simulink model "control1_flatness"  (R2023b)
settings: Solver=VariableStepAuto  StartTime=0.0  StopTime=8  RelTol=1e-3
values from neighbouring files (symbols this model uses):
  d = obs_r+threshold    (= 0.3)    [main.m]
  damping_coeff = 1/sqrt(2)    [main.m]
  initial_position = [0,r]    [main.m]
  natural_frequency = 10    [main.m]
  obs_r = 0.1    [main.m]
  obs_x = [20]    [main.m]
  obs_y = [20]    [main.m]
  parking_position = [0,0]    [main.m]
  r = 1    [main.m]
  T = 2*pi    (= 6.28318530718)    [main.m]
  t_values = 0:dt:T*1.1    [main.m]
  threshold = 0.2    [main.m]
(part 2 of 3)

== system control1_flatness/Trajectory generator/Trajectory generator and obstacle detection2/Subsystem3 ==
  Enable : EnablePort
  Clock1 : Clock
  Constant3 : Constant  Value=t_values
  Data Store Read : DataStoreRead  DataStoreName=iteration  IndexOptions=Index vector (dialog)  Indices=1  OutputSizes=1
  Data Store Read11 : DataStoreRead  DataStoreName=trajectory_x  IndexOptions=Index vector (dialog)  Indices=1  OutputSizes=1
  Data Store Read12 : DataStoreRead  DataStoreName=trajectory_y  IndexOptions=Index vector (dialog)  Indices=1  OutputSizes=1
  Data Store Read13 : DataStoreRead  DataStoreName=v_d_array  IndexOptions=Index vector (dialog)  Indices=1  OutputSizes=1
  Data Store Read14 : DataStoreRead  DataStoreName=omega_d_array  IndexOptions=Index vector (dialog)  Indices=1  OutputSizes=1
  Data Store Read15 : DataStoreRead  DataStoreName=theta_d_array  IndexOptions=Index vector (dialog)  Indices=1  OutputSizes=1
  Data Store Write : DataStoreWrite  DataStoreName=iteration  IndexOptions=Index vector (dialog)  Indices=1  OutputSizes=1
  Triggered Subsystem : Subsystem  TreatAsAtomicUnit=on
  x_d : Outport
  y_d : Outport  Port=2
  v_d : Outport  Port=3
  omega_d : Outport  Port=4
  theta_d : Outport  Port=5
  new_i : Outport  Port=6
  wires:
  Triggered Subsystem/3(v_d) -> v_d/1
  Triggered Subsystem/1(x_d) -> x_d/1
  Triggered Subsystem/2(y_d) -> y_d/1
  Data Store Read12/1 -> Triggered Subsystem/4(trajectory_y)
  Triggered Subsystem/4(omega_d) -> omega_d/1
  Data Store Read15/1 -> Triggered Subsystem/7(theta_d_array)
  Data Store Read14/1 -> Triggered Subsystem/6(omega_d_array)
  Data Store Read11/1 -> Triggered Subsystem/3(trajectory_x)
  Data Store Read13/1 -> Triggered Subsystem/5(v_d_array)
  Triggered Subsystem/5(theta_d) -> theta_d/1
  Clock1/1 -> Triggered Subsystem/1(t)
  Constant3/1 -> Triggered Subsystem/2(t_values)
  Data Store Read/1 -> Triggered Subsystem/8(Input)
  Triggered Subsystem/6(new_i) -> Data Store Write/1, new_i/1

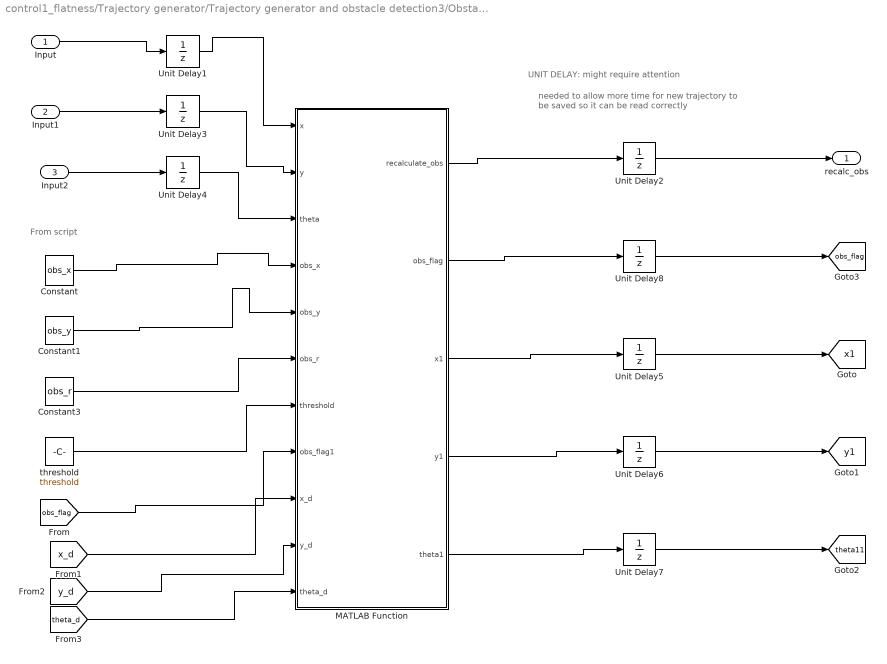
== system control1_flatness/Trajectory generator/Trajectory generator and obstacle detection3/Obstacle Detection ==
  note: UNIT DELAY: might require attention
  note: needed to allow more time for new trajectory to be saved
      | so it can be read correctly
  note: From script
  Input : Inport
  Input1 : Inport  Port=2
  Input2 : Inport  Port=3
  Constant : Constant  Value=obs_x
  Constant1 : Constant  Value=obs_y
  Constant3 : Constant  Value=obs_r
  MATLAB Function : MATLAB Function  TreatAsAtomicUnit=on
  Unit Delay{1..8} (8 alike) : UnitDelay  SampleTime=0.001  HasFrameUpgradeWarning=on
  threshold : Constant  Value=threshold
  recalc_obs : Outport
  tag scope: obs_flag=global, theta11=global, x1=global, y1=global
  wires:
  Constant/1 -> MATLAB Function/4(obs_x)
  Constant1/1 -> MATLAB Function/5(obs_y)
  Constant3/1 -> MATLAB Function/6(obs_r)
  threshold/1 -> MATLAB Function/7(threshold)
  [obs_flag] -> MATLAB Function/8(obs_flag1)
  MATLAB Function/2(obs_flag) -> Unit Delay8/1
  MATLAB Function/1(recalculate_obs) -> Unit Delay2/1
  Input/1 -> Unit Delay1/1
  Input1/1 -> Unit Delay3/1
  Unit Delay2/1 -> recalc_obs/1
  Unit Delay1/1 -> MATLAB Function/1(x)
  Unit Delay3/1 -> MATLAB Function/2(y)
  Input2/1 -> Unit Delay4/1
  Unit Delay4/1 -> MATLAB Function/3(theta)
  MATLAB Function/3(x1) -> Unit Delay5/1
  Unit Delay5/1 -> [x1]
  MATLAB Function/4(y1) -> Unit Delay6/1
  Unit Delay6/1 -> [y1]
  MATLAB Function/5(theta1) -> Unit Delay7/1
  Unit Delay7/1 -> [theta11]
  Unit Delay8/1 -> [obs_flag]
  [x_d] -> MATLAB Function/9(x_d)
  [y_d] -> MATLAB Function/10(y_d)
  [theta_d] -> MATLAB Function/11(theta_d)

== system control1_flatness/Trajectory generator/Trajectory generator and obstacle detection3/Subsystem1 ==
  recalc_obs : Inport
  theta : Inport  Port=2
  r : Inport  Port=3
  t_values : Inport  Port=4
  T : Inport  Port=5
  d : Inport  Port=6
  blending : Inport  Port=7
  old_traj_x : Inport  Port=8
  old_traj_y : Inport  Port=9
  xd : Inport  Port=10
  yd : Inport  Port=11
  Enable : EnablePort
  Whole trajectory calculation + flatness : MATLAB Function  TreatAsAtomicUnit=on
  recalculate : Outport
  recalculate_obs : Outport  Port=2
  trajectory_x : Outport  Port=3
  trajectory_y : Outport  Port=4
  v_d_array : Outport  Port=5
  omega_d_array : Outport  Port=6
  theta_d_array : Outport  Port=7
  wires:
  r/1 -> Whole trajectory calculation + flatness/1(r)
  Whole trajectory calculation + flatness/6(recalculate) -> recalculate/1
  t_values/1 -> Whole trajectory calculation + flatness/2(t_values)
  recalc_obs/1 -> Whole trajectory calculation + flatness/4(recalculate_obs)
  theta/1 -> Whole trajectory calculation + flatness/7(theta11)
  d/1 -> Whole trajectory calculation + flatness/5(d)
  Whole trajectory calculation + flatness/1(trajectory_x) -> trajectory_x/1
  Whole trajectory calculation + flatness/2(trajectory_y) -> trajectory_y/1
  Whole trajectory calculation + flatness/3(v_d_array) -> v_d_array/1
  Whole trajectory calculation + flatness/4(omega_d_array) -> omega_d_array/1
  Whole trajectory calculation + flatness/5(theta_d_array) -> theta_d_array/1
  T/1 -> Whole trajectory calculation + flatness/3(T)
  Whole trajectory calculation + flatness/7(recalculate_obs1) -> recalculate_obs/1
  blending/1 -> Whole trajectory calculation + flatness/6(blending)
  old_traj_x/1 -> Whole trajectory calculation + flatness/10(old_trajectory_x)
  old_traj_y/1 -> Whole trajectory calculation + flatness/11(old_trajectory_y)
  xd/1 -> Whole trajectory calculation + flatness/8(xd)
  yd/1 -> Whole trajectory calculation + flatness/9(yd)

== system control1_flatness/Trajectory generator/Trajectory generator and obstacle detection3/Subsystem3 ==
  Enable : EnablePort
  Clock1 : Clock
  Constant3 : Constant  Value=t_values
  Data Store Read : DataStoreRead  DataStoreName=iteration  IndexOptions=Index vector (dialog)  Indices=1  OutputSizes=1
  Data Store Read11 : DataStoreRead  DataStoreName=trajectory_x  IndexOptions=Index vector (dialog)  Indices=1  OutputSizes=1
  Data Store Read12 : DataStoreRead  DataStoreName=trajectory_y  IndexOptions=Index vector (dialog)  Indices=1  OutputSizes=1
  Data Store Read13 : DataStoreRead  DataStoreName=v_d_array  IndexOptions=Index vector (dialog)  Indices=1  OutputSizes=1
  Data Store Read14 : DataStoreRead  DataStoreName=omega_d_array  IndexOptions=Index vector (dialog)  Indices=1  OutputSizes=1
  Data Store Read15 : DataStoreRead  DataStoreName=theta_d_array  IndexOptions=Index vector (dialog)  Indices=1  OutputSizes=1
  Data Store Write : DataStoreWrite  DataStoreName=iteration  IndexOptions=Index vector (dialog)  Indices=1  OutputSizes=1
  Triggered Subsystem : Subsystem  TreatAsAtomicUnit=on
  x_d : Outport
  y_d : Outport  Port=2
  v_d : Outport  Port=3
  omega_d : Outport  Port=4
  theta_d : Outport  Port=5
  new_i : Outport  Port=6
  wires:
  Triggered Subsystem/3(v_d) -> v_d/1
  Triggered Subsystem/1(x_d) -> x_d/1
  Triggered Subsystem/2(y_d) -> y_d/1
  Data Store Read12/1 -> Triggered Subsystem/4(trajectory_y)
  Triggered Subsystem/4(omega_d) -> omega_d/1
  Data Store Read15/1 -> Triggered Subsystem/7(theta_d_array)
  Data Store Read14/1 -> Triggered Subsystem/6(omega_d_array)
  Data Store Read11/1 -> Triggered Subsystem/3(trajectory_x)
  Data Store Read13/1 -> Triggered Subsystem/5(v_d_array)
  Triggered Subsystem/5(theta_d) -> theta_d/1
  Clock1/1 -> Triggered Subsystem/1(t)
  Constant3/1 -> Triggered Subsystem/2(t_values)
  Data Store Read/1 -> Triggered Subsystem/8(Input)
  Triggered Subsystem/6(new_i) -> Data Store Write/1, new_i/1

== system control1_flatness/Trajectory generator/Trajectory generator and obstacle detection/Subsystem3/Triggered Subsystem ==
  t : Inport
  t_values : Inport  Port=2
  trajectory_x : Inport  Port=3
  trajectory_y : Inport  Port=4
  v_d_array : Inport  Port=5
  omega_d_array : Inport  Port=6
  theta_d_array : Inport  Port=7
  Input : Inport  Port=8
  MATLAB Function1 : MATLAB Function  TreatAsAtomicUnit=on
  x_d : Outport
  y_d : Outport  Port=2
  v_d : Outport  Port=3
  omega_d : Outport  Port=4
  theta_d : Outport  Port=5
  new_i : Outport  Port=6
  wires:
  trajectory_x/1 -> MATLAB Function1/3(trajectory_x)
  trajectory_y/1 -> MATLAB Function1/4(trajectory_y)
  MATLAB Function1/1(x_d) -> x_d/1
  MATLAB Function1/2(y_d) -> y_d/1
  t/1 -> MATLAB Function1/1(t)
  t_values/1 -> MATLAB Function1/2(t_values)
  v_d_array/1 -> MATLAB Function1/5(v_d_array)
  omega_d_array/1 -> MATLAB Function1/6(omega_d_array)
  theta_d_array/1 -> MATLAB Function1/7(theta_d_array)
  MATLAB Function1/3(v_d) -> v_d/1
  MATLAB Function1/4(omega_d) -> omega_d/1
  MATLAB Function1/5(theta_d) -> theta_d/1
  Input/1 -> MATLAB Function1/8(i)
  MATLAB Function1/6(new_i) -> new_i/1

== system control1_flatness/Trajectory generator/Trajectory generator and obstacle detection1/Subsystem3/Triggered Subsystem ==
  t : Inport
  t_values : Inport  Port=2
  trajectory_x : Inport  Port=3
  trajectory_y : Inport  Port=4
  v_d_array : Inport  Port=5
  omega_d_array : Inport  Port=6
  theta_d_array : Inport  Port=7
  Input : Inport  Port=8
  MATLAB Function1 : MATLAB Function  TreatAsAtomicUnit=on
  x_d : Outport
  y_d : Outport  Port=2
  v_d : Outport  Port=3
  omega_d : Outport  Port=4
  theta_d : Outport  Port=5
  new_i : Outport  Port=6
  wires:
  trajectory_x/1 -> MATLAB Function1/3(trajectory_x)
  trajectory_y/1 -> MATLAB Function1/4(trajectory_y)
  MATLAB Function1/1(x_d) -> x_d/1
  MATLAB Function1/2(y_d) -> y_d/1
  t/1 -> MATLAB Function1/1(t)
  t_values/1 -> MATLAB Function1/2(t_values)
  v_d_array/1 -> MATLAB Function1/5(v_d_array)
  omega_d_array/1 -> MATLAB Function1/6(omega_d_array)
  theta_d_array/1 -> MATLAB Function1/7(theta_d_array)
  MATLAB Function1/3(v_d) -> v_d/1
  MATLAB Function1/4(omega_d) -> omega_d/1
  MATLAB Function1/5(theta_d) -> theta_d/1
  Input/1 -> MATLAB Function1/8(i)
  MATLAB Function1/6(new_i) -> new_i/1

== system control1_flatness/Trajectory generator/Trajectory generator and obstacle detection2/Subsystem3/Triggered Subsystem ==
  t : Inport
  t_values : Inport  Port=2
  trajectory_x : Inport  Port=3
  trajectory_y : Inport  Port=4
  v_d_array : Inport  Port=5
  omega_d_array : Inport  Port=6
  theta_d_array : Inport  Port=7
  Input : Inport  Port=8
  MATLAB Function1 : MATLAB Function  TreatAsAtomicUnit=on
  x_d : Outport
  y_d : Outport  Port=2
  v_d : Outport  Port=3
  omega_d : Outport  Port=4
  theta_d : Outport  Port=5
  new_i : Outport  Port=6
  wires:
  trajectory_x/1 -> MATLAB Function1/3(trajectory_x)
  trajectory_y/1 -> MATLAB Function1/4(trajectory_y)
  MATLAB Function1/1(x_d) -> x_d/1
  MATLAB Function1/2(y_d) -> y_d/1
  t/1 -> MATLAB Function1/1(t)
  t_values/1 -> MATLAB Function1/2(t_values)
  v_d_array/1 -> MATLAB Function1/5(v_d_array)
  omega_d_array/1 -> MATLAB Function1/6(omega_d_array)
  theta_d_array/1 -> MATLAB Function1/7(theta_d_array)
  MATLAB Function1/3(v_d) -> v_d/1
  MATLAB Function1/4(omega_d) -> omega_d/1
  MATLAB Function1/5(theta_d) -> theta_d/1
  Input/1 -> MATLAB Function1/8(i)
  MATLAB Function1/6(new_i) -> new_i/1

== system control1_flatness/Trajectory generator/Trajectory generator and obstacle detection3/Subsystem3/Triggered Subsystem ==
  t : Inport
  t_values : Inport  Port=2
  trajectory_x : Inport  Port=3
  trajectory_y : Inport  Port=4
  v_d_array : Inport  Port=5
  omega_d_array : Inport  Port=6
  theta_d_array : Inport  Port=7
  Input : Inport  Port=8
  MATLAB Function1 : MATLAB Function  TreatAsAtomicUnit=on
  x_d : Outport
  y_d : Outport  Port=2
  v_d : Outport  Port=3
  omega_d : Outport  Port=4
  theta_d : Outport  Port=5
  new_i : Outport  Port=6
  wires:
  trajectory_x/1 -> MATLAB Function1/3(trajectory_x)
  trajectory_y/1 -> MATLAB Function1/4(trajectory_y)
  MATLAB Function1/1(x_d) -> x_d/1
  MATLAB Function1/2(y_d) -> y_d/1
  t/1 -> MATLAB Function1/1(t)
  t_values/1 -> MATLAB Function1/2(t_values)
  v_d_array/1 -> MATLAB Function1/5(v_d_array)
  omega_d_array/1 -> MATLAB Function1/6(omega_d_array)
  theta_d_array/1 -> MATLAB Function1/7(theta_d_array)
  MATLAB Function1/3(v_d) -> v_d/1
  MATLAB Function1/4(omega_d) -> omega_d/1
  MATLAB Function1/5(theta_d) -> theta_d/1
  Input/1 -> MATLAB Function1/8(i)
  MATLAB Function1/6(new_i) -> new_i/1

== matlab function control1_flatness/Trajectory generator/Trajectory generator and obstacle detection2/Obstacle Detection/MATLAB Function ==
  data: x input; y input; theta input; obs_x input; obs_y input; obs_r input; threshold input; obs_flag1 input; recalculate_obs output; obs_flag output; x1 output; y1 output; theta1 output; x_d input; y_d input; theta_d input
function [recalculate_obs, obs_flag, x1, y1, theta1] = distance_sensor(x, y, theta, obs_x, obs_y, obs_r, threshold, obs_flag1, x_d, y_d, theta_d)
% input:
% x, y: Unicycle's position
% for fixed obstacle
% obs_x, obs_y: Obstacle's position
% obs_r: Obstacle's radius
% threshold: Detection range

% Output:
obs_flag = 0;
for i = 1:length(obs_x)
    % Compute Euclidean distance to the obstacle
    distance = sqrt((x - obs_x(i))^2 + (y - obs_y(i))^2);
    
    % Check if the obstacle is within the detection range and within ±30° of theta
    if (distance <= (obs_r + threshold))
        angle_to_obstacle = atan2(obs_y(i) - y, obs_x(i) - x);
        % Compute the angle difference (normalize to [-pi, pi] range)
        angle_diff=mod(abs(angle_to_obstacle - theta), 2*pi);
        if(abs(angle_diff) <= pi/4)
            obs_flag = 1; % Obstacle detected in front sector
            break;
        else
           obs_flag = 0; 
        end
    end
end
    
if obs_flag && ~obs_flag1
    % Obstacle detected for the first time, trigger recalculation
    recalculate_obs = 1;
else
    % Either no obstacle or already recalculated
    recalculate_obs = 0;
end
x1 = x_d;
y1 = y_d;
theta1 = theta_d;

== matlab function control1_flatness/Trajectory generator/Trajectory generator and obstacle detection2/Subsystem1/Whole trajectory calculation + flatness ==
  data: r input; trajectory_x output; t_values input; T input; trajectory_y output; v_d_array output; omega_d_array output; theta_d_array output; recalculate output; recalculate_obs input; d input; blending input; theta11 input; xd input; yd input; recalculate_obs1 output; old_trajectory_x input; old_trajectory_y input
function [trajectory_x, trajectory_y, v_d_array, omega_d_array, theta_d_array, recalculate,recalculate_obs1]  = fcn( r, t_values,T, recalculate_obs,d, blending, theta11, xd, yd,old_trajectory_x, old_trajectory_y)
    if(~recalculate_obs)
        trajectory_x = zeros(length(t_values),1);
        trajectory_y = ones(length(t_values),1);
    
         for i = 1:length(t_values)
              t = t_values(i);
              if(t<T)
                  trajectory_x(i)= r*cos(t)-1;
                  trajectory_y(i) = r*sin(2*t)/2+1;
              else
                  trajectory_x(i)= r*cos(T)-1;
                  trajectory_y(i) = r*sin(2*T)/2+1;
              end
          end   
    else
        % Obstacle was detected: in the point x, y with angle theta
        center_1 = [-0.4,1];
        center_2 = [-1.6,1];
        % Loading previous version of the trajectory 
        % to avoid additional and useless computations of
        % previous desired path
        trajectory_x = old_trajectory_x;
        trajectory_y = old_trajectory_y;
        x1 = xd;
        y1 = yd;
        points = [trajectory_x,trajectory_y];
        [~, start_idx] = min(vecnorm(points - [x1,y1], 2, 2));

        theta1 = -theta11+pi/2;  % Adjusting the angle to get the angle from vertical axis (theta11 is wrt horisontal axis)

        % Estimate the obstacle location
        theta_range = linspace(theta1 - pi/4, theta1 + pi/4, 300);
        x_arc = x1 + d * sin(theta_range);
        y_arc = y1 + d * cos(theta_range);

        % Loop through the trajectory points to check for intersections

        obs_x = x1;
        obs_y = y1;
        obs_idx = start_idx;
        for i = start_idx:length(trajectory_x) - 1
            x_traj_seg = [trajectory_x(i), trajectory_x(i + 1)];
            y_traj_seg = [trajectory_y(i), trajectory_y(i + 1)];
            
            for j = 1:length(x_arc) - 1
                x_arc_seg = [x_arc(j), x_arc(j + 1)];
                y_arc_seg = [y_arc(j), y_arc(j + 1)];
                
                % Check if the two segments intersect
                [intersects, ix, iy] = segmentIntersection(x_traj_seg, y_traj_seg, x_arc_seg, y_arc_seg);
        
                if intersects
                    % Intersection found, assign coordinates
                    obs_x = ix;
                    obs_y = iy;
                    obs_idx = i;
                    break; % Exit the loop once intersection is found
                end
             end
            if obs_x ~= x1
                break; 
            end
        end

        % -- > Finding the point where the obstacle avoidance trajectory should 
        % be finished, point from which the robot should continue on
        % the regular trajectory.Creating a circle of radius d, with the 
        % center in [center_obs_x, center_obs_y].
        % After that, finding an intersection of that circle with the 
        % previous trajectory.

        theta_values = linspace(0, 2*pi, 500);
        x_circle = obs_x + d * cos(theta_values);
        y_circle = obs_y + d * sin(theta_values);

        % Loop through the trajectory points to check for intersections

        x2 = x1;
        y2 = y1;
        end_idx_trajectory = obs_idx;
        end_idx_circle = 1;

        for i = obs_idx:length(trajectory_x) - 1
            x_traj_seg = [trajectory_x(i), trajectory_x(i + 1)];
            y_traj_seg = [trajectory_y(i), trajectory_y(i + 1)];
            
            for j = 1:length(x_circle) - 1
                x_circle_seg = [x_circle(j), x_circle(j + 1)];
                y_circle_seg = [y_circle(j), y_circle(j + 1)];
                
                % Check if the two segments intersect
                [intersects, ix, iy] = segmentIntersection(x_traj_seg, y_traj_seg, x_circle_seg, y_circle_seg);
        
                if intersects
                    % Intersection found, assign coordinates
                    x2 = ix;
                    y2 = iy;
                    end_idx_trajectory = i;
                    end_idx_circle = j;
                    break; 
                end
            end
            if x2 ~= x1, break; end
        end

        % --> Finding the longer arc of the circle around obstacle
        % This will be the desired obstacle avoidance path
        points = [x_circle' y_circle']; % Nx2 array
        [~, idx1] = min(vecnorm(points - [x1,y1], 2, 2));
        idx2 = end_idx_circle;
        
        if idx1 < idx2
            arc1 = points(idx1:idx2, :);       
            arc2 = [points(idx2:end, :); points(1:idx1, :)];
        else
            arc1 = points(idx2:idx1, :);       
            arc2 = [points(idx1:end, :); points(1:idx2, :)];
        end

        idx_point1 = floor(size(arc1,1)/2);
        idx_point2 = floor(size(arc2,1)/2);


        distance1 = (x1-center_1(1))^2+(y1-center_1(2))^2;
        distance2 = (x1-center_2(1))^2+(y1-center_2(2))^2;

        if(distance1<distance2)
            distance1 = (arc1(idx_point1,1)-center_1(1))^2+(arc1(idx_point1,2)-center_1(2))^2;
            distance2 = (arc2(idx_point2,1)-center_1(1))^2+(arc2(idx_point2,2)-center_1(2))^2;
        else
            distance1 = (arc1(idx_point1,1)-center_2(1))^2+(arc1(idx_point1,2)-center_2(2))^2;
            distance2 = (arc2(idx_point2,1)-center_2(1))^2+(arc2(idx_point2,2)-center_2(2))^2;
        end

        if distance1>distance2
            chosen_arc = arc1;
        else
            chosen_arc = arc2;
        end

        % Reverse if needed
        if(abs(chosen_arc(1,1)-x1)>abs(chosen_arc(1,1)-x2))
            chosen_arc = flip(chosen_arc);
        end

        % --> Creating a new trajectory
        idx1 = start_idx;
        idx2 = end_idx_trajectory;
        % Change of the trajectory is allowed if the ordering is okay
        % first indexwise is the point of detection and then the obstacle
        % (should always be satisfied)
        if(idx1<idx2 && t_values(idx2)<T)

            n_points = idx2 - idx1 + 1;
            total_points = size(chosen_arc,1);
            indices = round(linspace(1, total_points, n_points));
            % Smoothly blend the two trajectories if needed
            trajectory_avoid_x = chosen_arc(indices,1);
            trajectory_avoid_y = chosen_arc(indices,2);
            trajectory_old_x = trajectory_x(idx1:idx2);
            trajectory_old_y = trajectory_y(idx1:idx2);

            trajectory_x(idx1:idx2) = blending*trajectory_avoid_x + (1-blending)*trajectory_old_x;
            trajectory_y(idx1:idx2) = blending*trajectory_avoid_y + (1-blending)*trajectory_old_y;

        end
    end

    recalculate_obs1 = 0;
    recalculate = 0;


    dt = t_values(2) - t_values(1);

    %  Derivatives
    dx_d = gradient(trajectory_x, dt);
    dy_d = gradient(trajectory_y, dt);
    ddx_d = gradient(dx_d, dt);
    ddy_d = gradient(dy_d, dt);
    
    v_d_array = sqrt(dx_d.^2 + dy_d.^2);
    omega_d_array = (ddy_d .* dx_d - ddx_d .* dy_d) ./ ((dx_d.^2 + dy_d.^2)+eps);
    theta_d_array=atan2(dy_d,dx_d);

end

== matlab function control1_flatness/Regulation task: controller and model /Cartesian Controller/Controller ==
  data: v output; omega output; x input; y input; theta input
function [v, omega]= fcn(x, y, theta)
k1 =0.5;
k2 =30;
v = k1*(-x*cos(theta)-y*sin(theta));
omega = k2*(atan2(y,x)+pi-theta);

== matlab function control1_flatness/Trajectory generator/Trajectory generator and obstacle detection/Obstacle Detection/MATLAB Function ==
  data: x input; y input; theta input; obs_x input; obs_y input; obs_r input; threshold input; obs_flag1 input; recalculate_obs output; obs_flag output; x1 output; y1 output; theta1 output
function [recalculate_obs, obs_flag, x1, y1, theta1] = distance_sensor(x, y, theta, obs_x, obs_y, obs_r, threshold, obs_flag1)
% input:
% x, y: Unicycle's position
% for fixed obstacle
% obs_x, obs_y: Obstacle's position
% obs_r: Obstacle's radius
% threshold: Detection range

% Output:
obs_flag = 0;
for i = 1:length(obs_x)
    % Compute Euclidean distance to the obstacle
    distance = sqrt((x - obs_x(i))^2 + (y - obs_y(i))^2);
    
    % Check if the obstacle is within the detection range and within ±30° of theta
    if (distance <= (obs_r + threshold))
        angle_to_obstacle = atan2(obs_y(i) - y, obs_x(i) - x);
        % Compute the angle difference (normalize to [-pi, pi] range)
        %angle_diff = mod(angle_to_obstacle + theta, 2*pi)-pi
        angle_diff=mod(abs(angle_to_obstacle - theta), 2*pi);
        if(abs(angle_diff) <= pi/4)
            obs_flag = 1; % Obstacle detected in front sector
            break;
        else
           obs_flag = 0; 
        end
    end
end
    
if obs_flag && ~obs_flag1
    % Obstacle detected for the first time, trigger recalculation
    recalculate_obs = 1;
else
    % Either no obstacle or already recalculated
    recalculate_obs = 0;
end
x1 = x;
y1 = y;
theta1 = theta;

== matlab function control1_flatness/Trajectory generator/Trajectory generator and obstacle detection2/Subsystem3/Triggered Subsystem/MATLAB Function1 ==
  data: t input; t_values input; trajectory_x input; x_d output; trajectory_y input; y_d output; v_d output; omega_d output; theta_d output; v_d_array input; omega_d_array input; theta_d_array input; i input; new_i output
function [x_d, y_d, v_d, omega_d, theta_d, new_i] = fcn(t, t_values, trajectory_x, trajectory_y, v_d_array, omega_d_array, theta_d_array,i)

    % When the block is not enabled (on the start),this is used to give initial position
    if (i==0)
        new_i=1;
    else
        new_i =i;
    end

    [~, idx] = min(abs(t_values - t));  % closest index to current time
    if(t>t_values(end))
        idx = length(t_values);
    end
    % Position
    x_d = trajectory_x(idx);  
    y_d = trajectory_y(idx);

    % Flatness
    v_d = v_d_array(idx);  
    omega_d = omega_d_array(idx);
    theta_d = theta_d_array(idx);

== matlab function control1_flatness/Trajectory generator/Trajectory generator and obstacle detection3/MATLAB Function ==
  data: initial_position input; x1 input; y1 input; v1 input; omega1 input; theta1 input; i input; x output; y output; v output; omega output; theta output
function [x,y,v,omega,theta] = fcn(initial_position, x1,y1,v1, omega1, theta1,i)

if(i == 0)
    x = initial_position(1);
    y = initial_position(2);
    v = 0;
    omega = 0;
    theta=0;
else
    x = x1;
    y = y1;
    v = v1;
    omega = omega1;
    theta=theta1;
end

== matlab function control1_flatness/Trajectory generator/Trajectory generator and obstacle detection/Subsystem3/Triggered Subsystem/MATLAB Function1 ==
  data: t input; t_values input; trajectory_x input; x_d output; trajectory_y input; y_d output; v_d output; omega_d output; theta_d output; v_d_array input; omega_d_array input; theta_d_array input; i input; new_i output
function [x_d, y_d, v_d, omega_d, theta_d, new_i] = fcn(t, t_values, trajectory_x, trajectory_y, v_d_array, omega_d_array, theta_d_array,i)

    % When the block is not enabled (on the start),this is used to give initial position
    if (i==0)
        new_i=1;
    else
        new_i =i;
    end

    [~, idx] = min(abs(t_values - t));  % closest index to current time
    if(t>t_values(end))
        idx = length(t_values);
    end
    % Position
    x_d = trajectory_x(idx);  
    y_d = trajectory_y(idx);

    % Flatness
    v_d = v_d_array(idx);  
    omega_d = omega_d_array(idx);
    theta_d = theta_d_array(idx);

== matlab function control1_flatness/Trajectory generator/Trajectory generator and obstacle detection3/Obstacle Detection/MATLAB Function ==
  data: x input; y input; theta input; obs_x input; obs_y input; obs_r input; threshold input; obs_flag1 input; recalculate_obs output; obs_flag output; x1 output; y1 output; theta1 output; x_d input; y_d input; theta_d input
function [recalculate_obs, obs_flag, x1, y1, theta1] = distance_sensor(x, y, theta, obs_x, obs_y, obs_r, threshold, obs_flag1, x_d, y_d, theta_d)
% input:
% x, y: Unicycle's position
% for fixed obstacle
% obs_x, obs_y: Obstacle's position
% obs_r: Obstacle's radius
% threshold: Detection range

% Output:
obs_flag = 0;
for i = 1:length(obs_x)
    % Compute Euclidean distance to the obstacle
    distance = sqrt((x - obs_x(i))^2 + (y - obs_y(i))^2);
    
    % Check if the obstacle is within the detection range and within ±30° of theta
    if (distance <= (obs_r + threshold))
        angle_to_obstacle = atan2(obs_y(i) - y, obs_x(i) - x);
        % Compute the angle difference (normalize to [-pi, pi] range)
        angle_diff=mod(abs(angle_to_obstacle - theta), 2*pi);
        if(abs(angle_diff) <= pi/4)
            obs_flag = 1; % Obstacle detected in front sector
            break;
        else
           obs_flag = 0; 
        end
    end
end
    
if obs_flag && ~obs_flag1
    % Obstacle detected for the first time, trigger recalculation
    recalculate_obs = 1;
else
    % Either no obstacle or already recalculated
    recalculate_obs = 0;
end
x1 = x_d;
y1 = y_d;
theta1 = theta_d;

== matlab function control1_flatness/Trajectory generator/Trajectory generator and obstacle detection3/Subsystem1/Whole trajectory calculation + flatness ==
  data: r input; trajectory_x output; t_values input; T input; trajectory_y output; v_d_array output; omega_d_array output; theta_d_array output; recalculate output; recalculate_obs input; d input; blending input; theta11 input; xd input; yd input; recalculate_obs1 output; old_trajectory_x input; old_trajectory_y input
function [trajectory_x, trajectory_y, v_d_array, omega_d_array, theta_d_array, recalculate,recalculate_obs1]  = fcn( r, t_values,T, recalculate_obs,d, blending, theta11, xd, yd,old_trajectory_x, old_trajectory_y)
    if(~recalculate_obs)
        trajectory_x = zeros(length(t_values), 1);
        trajectory_y = ones(length(t_values), 1);
        % Triangle parameters
        W = 4;  % Base width
        H = 3;  % Height
        x0 = 0;  % Starting x-coordinate
        y0 = 1;  % Starting y-coordinate

        for i = 1:length(t_values)
            t = t_values(i);
            
            if t < T/3
                % Move up diagonally (first leg)
                trajectory_x(i) = x0 + (W/2) * (t / (T/3));
                trajectory_y(i) = y0 + H * (t / (T/3));
                
            elseif t < 2*T/3
                % Move down diagonally (second leg)
                trajectory_x(i) = x0 + (W/2) + (W/2) * ((t - T/3) / (T/3));
                trajectory_y(i) = y0 + H - H * ((t - T/3) / (T/3));
                
            elseif t<T
                % Move horizontally back to start (third leg)
                trajectory_x(i) = x0 + W - W * ((t - 2*T/3) / (T/3));
                trajectory_y(i) = y0;
            else
                trajectory_x(i) = x0;
                trajectory_y(i) = y0;
            end
        end

    else
        % Obstacle was detected: in the point x, y with angle theta
        W = 4;  % Base width
        H = 3;  % Height
        x0 = 0;  % Starting x-coordinate
        y0 = 1;  % Starting y-coordinate
        center_trajectory = [x0+W/2, y0+H/2];
        % Loading previous version of the trajectory 
        % to avoid additional and useless computations of
        % previous desired path
        trajectory_x = old_trajectory_x;
        trajectory_y = old_trajectory_y;
        x1 = xd;
        y1 = yd;
        points = [trajectory_x,trajectory_y];
        [~, start_idx] = min(vecnorm(points - [x1,y1], 2, 2));

        theta1 = -theta11+pi/2;  % Adjusting the angle to get the anglefrom vertical axis (theta11 is wrt horisontal axis)

        % Estimate the obstacle location
        theta_range = linspace(theta1 - pi/4, theta1 + pi/4, 300);
        x_arc = x1 + d * sin(theta_range);
        y_arc = y1 + d * cos(theta_range);



        % Loop through the trajectory points to check for intersections

        obs_x = x1;
        obs_y = y1;
        obs_idx = start_idx;
        for i = start_idx:length(trajectory_x) - 1
            x_traj_seg = [trajectory_x(i), trajectory_x(i + 1)];
            y_traj_seg = [trajectory_y(i), trajectory_y(i + 1)];
            
            for j = 1:length(x_arc) - 1
                x_arc_seg = [x_arc(j), x_arc(j + 1)];
                y_arc_seg = [y_arc(j), y_arc(j + 1)];
                
                % Check if the two segments intersect
                [intersects, ix, iy] = segmentIntersection(x_traj_seg, y_traj_seg, x_arc_seg, y_arc_seg);
        
                if intersects
                    % Intersection found, assign coordinates
                    obs_x = ix;
                    obs_y = iy;
                    obs_idx = i;
                    break; % Exit the loop once intersection is found
                end
             end
            if obs_x ~= x1
                break; 
            end
        end

        % -- > Finding the point where the obstacle avoidance trajectory should 
        % be finished, point from which the robot should continue on
        % the regular trajectory.Creating a circle of radius d, with the 
        % center in [center_obs_x, center_obs_y].
        % After that, finding an intersection of that circle with the 
        % previous trajectory.
    
        theta_values = linspace(0, 2*pi, 500);
        x_circle = obs_x + d * cos(theta_values);
        y_circle = obs_y + d * sin(theta_values);

        % Loop through the trajectory points to check for intersections

        x2 = x1;
        y2 = y1;
        end_idx_trajectory = obs_idx;
        end_idx_circle = 1;

        for i = obs_idx:length(trajectory_x) - 1
            x_traj_seg = [trajectory_x(i), trajectory_x(i + 1)];
            y_traj_seg = [trajectory_y(i), trajectory_y(i + 1)];
            
            for j = 1:length(x_circle) - 1
                x_circle_seg = [x_circle(j), x_circle(j + 1)];
                y_circle_seg = [y_circle(j), y_circle(j + 1)];
                
                % Check if the two segments intersect
                [intersects, ix, iy] = segmentIntersection(x_traj_seg, y_traj_seg, x_circle_seg, y_circle_seg);
        
                if intersects
                    % Intersection found, assign coordinates
                    x2 = ix;
                    y2 = iy;
                    end_idx_trajectory = i;
                    end_idx_circle = j;
                    break; 
                end
            end
            if x2 ~= x1, break; end
        end

        % --> Finding the longer arc of the circle around obstacle
        % This will be the desired obstacle avoidance path
        points = [x_circle' y_circle']; % Nx2 array
        [~, idx1] = min(vecnorm(points - [x1,y1], 2, 2));
        idx2 = end_idx_circle;
        
        if idx1 < idx2
            arc1 = points(idx1:idx2, :);       
            arc2 = [points(idx2:end, :); points(1:idx1, :)];
        else
            arc1 = points(idx2:idx1, :);       
            arc2 = [points(idx1:end, :); points(1:idx2, :)];
        end
        
        idx_point1 = floor(size(arc1,1)/2);
        idx_point2 = floor(size(arc2,1)/2);
        
        distance1 = (arc1(idx_point1,1)-center_trajectory(1))^2+(arc1(idx_point1,2)-center_trajectory(2))^2;
        distance2 =  (arc2(idx_point2,1)-center_trajectory(1))^2+(arc2(idx_point2,2)-center_trajectory(2))^2;
        
        if distance1>distance2
            longer_arc = arc1;
        else
            longer_arc = arc2;
        end
        % Reverse if needed
        if(abs(longer_arc(1,1)-x1)>abs(longer_arc(1,1)-x2))
            longer_arc = flip(longer_arc);
        end


        % --> Creating a new trajectory
        idx1 = start_idx;
        idx2 = end_idx_trajectory;
        % Change of the trajectory is allowed if the ordering is okay
        % first indexwise is the point of detection and then the obstacle
        % (should always be satisfied)
        if(idx1<idx2 && t_values(idx2)<T)

            n_points = idx2 - idx1 + 1;
            total_points = size(longer_arc,1);
            indices = round(linspace(1, total_points, n_points));
            % Smoothly blend the two trajectories if needed
            trajectory_avoid_x = longer_arc(indices,1);
            trajectory_avoid_y = longer_arc(indices,2);
            trajectory_old_x = trajectory_x(idx1:idx2);
            trajectory_old_y = trajectory_y(idx1:idx2);

            trajectory_x(idx1:idx2) = blending*trajectory_avoid_x + (1-blending)*trajectory_old_x;
            trajectory_y(idx1:idx2) = blending*trajectory_avoid_y + (1-blending)*trajectory_old_y;

        end
    end

    recalculate_obs1 = 0;
    recalculate = 0;


    dt = t_values(2) - t_values(1);

    %  Derivatives
    dx_d = gradient(trajectory_x, dt);
    dy_d = gradient(trajectory_y, dt);
    ddx_d = gradient(dx_d, dt);
    ddy_d = gradient(dy_d, dt);
    
    v_d_array = sqrt(dx_d.^2 + dy_d.^2);
    omega_d_array = (ddy_d .* dx_d - ddx_d .* dy_d) ./ ((dx_d.^2 + dy_d.^2)+eps);
    theta_d_array=atan2(dy_d,dx_d);

end

== matlab function control1_flatness/Output ==
  data: x1 input; y1 input; theta1 input; regulation_flag input; x_out output; x2 input; y2 input; theta2 input; y_out output; theta_out output
function [x_out, y_out, theta_out]  = fcn(x1, y1, theta1, regulation_flag, x2, y2, theta2)
if(regulation_flag==0)
    x_out = x1;
    y_out = y1;
    theta_out = theta1;

else
    x_out = x2;
    y_out = y2;
    theta_out = theta2;
  
end

== matlab function control1_flatness/Trajectory generator/Trajectory generator and obstacle detection3/Subsystem3/Triggered Subsystem/MATLAB Function1 ==
  data: t input; t_values input; trajectory_x input; x_d output; trajectory_y input; y_d output; v_d output; omega_d output; theta_d output; v_d_array input; omega_d_array input; theta_d_array input; i input; new_i output
function [x_d, y_d, v_d, omega_d, theta_d, new_i] = fcn(t, t_values, trajectory_x, trajectory_y, v_d_array, omega_d_array, theta_d_array,i)

    % When the block is not enabled (on the start),this is used to give initial position
    if (i==0)
        new_i=1;
    else
        new_i =i;
    end

    [~, idx] = min(abs(t_values - t));  % closest index to current time
    if(t>t_values(end))
        idx = length(t_values);
    end
    % Position
    x_d = trajectory_x(idx);  
    y_d = trajectory_y(idx);

    % Flatness
    v_d = v_d_array(idx);  
    omega_d = omega_d_array(idx);
    theta_d = theta_d_array(idx);

== matlab function control1_flatness/Regulation task: controller and model /Cartesian Controller/MATLAB Function2 ==
  data: v input; x_dot output; omega input; theta input; y_dot output; theta_dot output; reg_flag input; v_for_graph output; omega_for_graph output; v_not_regulation input; omega_not_regulation input
function [x_dot, y_dot, theta_dot, v_for_graph, omega_for_graph] = model(v, omega, theta,reg_flag, v_not_regulation, omega_not_regulation)
    if(reg_flag)
        x_dot=v.*cos(theta);
        y_dot=v.*sin(theta);
        theta_dot=omega;
        v_for_graph = v;
        omega_for_graph = omega;
    else
        x_dot=0;
        y_dot=0;
        theta_dot=0;
        v_for_graph = v_not_regulation;
        omega_for_graph = omega_not_regulation;
    end


end

== matlab function control1_flatness/Parked indication ==
  data: x input; parked_flag output; y input; e input
function parked_flag = fcn(x, y, e)
parked_flag = 0;
if(abs(x)<e && abs(y)<e)
    parked_flag=1;
end

== matlab function control1_flatness/Regulation task: controller and model /Controller with polar coordinates/Controller ==
  data: u output; omega output; gamma input; delta input
function [u, omega]= fcn(gamma, delta)
k1 = 0.5;
k2 = 2;
k3 = 1;

u = k1*cos(gamma);
omega = k2*gamma+k1*sin(gamma)*cos(gamma)*(gamma+k3*delta);

== matlab function control1_flatness/Regulation task: controller and model /Controller with polar coordinates/Transformation to Cartesian coordinates ==
  data: x output; rho input; y output; gamma input; delta input; theta output
function [x, y, theta] = fcn(rho, gamma, delta)
gamma1 = wrapToPi(gamma);
delta1 = wrapToPi(delta);

theta = delta1 - gamma1; 

x = -rho*cos(delta1);
y = -rho*sin(delta1);

== matlab function control1_flatness/Regulation task: controller and model /Controller with polar coordinates/Transformation to polar coordinates ==
  data: rho output; x input; gamma output; y input; theta input; delta output
function [rho, gamma, delta] = fcn(x, y, theta)

rho = sqrt(x^2+y^2);
gamma = wrapToPi(atan2(y, x) - theta + pi);
delta = wrapToPi(gamma + theta);

== matlab function control1_flatness/Regulation task: controller and model /Controller with polar coordinates/Unicycle model: polar coordinates ==
  data: rho input; gamma input; u input; rho_dot output; omega input; gamma_dot output; delta_dot output; regulation_flag input
function [rho_dot, gamma_dot, delta_dot] = model(rho, gamma, u, omega, regulation_flag)
if(regulation_flag)
    rho_dot = -u*rho*cos(gamma);
    gamma_dot = sin(gamma)*u-omega;
    delta_dot = sin(gamma)*u;
else
    rho_dot = 0;
    gamma_dot = 0;
    delta_dot = 0;
end

== matlab function control1_flatness/Regulation task: controller and model /Regulation controller choice ==
  data: x1 input; y1 input; theta1 input; controller_choice input; x_out output; x2 input; y2 input; theta2 input; y_out output; theta_out output
function [x_out, y_out, theta_out] = fcn(x1, y1, theta1, controller_choice, x2, y2, theta2 )
if(controller_choice==1)
    x_out = x1;
    y_out = y1;
    theta_out = theta1;
else
    x_out = x2;
    y_out = y2;
    theta_out = theta2;
end

== matlab function control1_flatness/Trajectory generator/Trajectory generator and obstacle detection1/MATLAB Function ==
  data: initial_position input; x1 input; y1 input; v1 input; omega1 input; theta1 input; i input; x output; y output; v output; omega output; theta output
function [x,y,v,omega,theta] = fcn(initial_position, x1,y1,v1, omega1, theta1,i)

if(i == 0)
    x = initial_position(1);
    y = initial_position(2);
    v = 0;
    omega = 0;
    theta=0;
else
    x = x1;
    y = y1;
    v = v1;
    omega = omega1;
    theta=theta1;
end

== matlab function control1_flatness/Trajectory generator/Trajectory generator and obstacle detection1/Obstacle Detection/MATLAB Function ==
  data: x input; y input; theta input; obs_x input; obs_y input; obs_r input; threshold input; obs_flag1 input; recalculate_obs output; obs_flag output; x1 output; y1 output; theta1 output; x_d input; y_d input; theta_d input
function [recalculate_obs, obs_flag, x1, y1, theta1] = distance_sensor(x, y, theta, obs_x, obs_y, obs_r, threshold, obs_flag1, x_d, y_d, theta_d)
% input:
% x, y: Unicycle's position
% for fixed obstacle
% obs_x, obs_y: Obstacle's position
% obs_r: Obstacle's radius
% threshold: Detection range

% Output:
obs_flag = 0;
for i = 1:length(obs_x)
    % Compute Euclidean distance to the obstacle
    distance = sqrt((x - obs_x(i))^2 + (y - obs_y(i))^2);
    
    % Check if the obstacle is within the detection range and within ±30° of theta
    if (distance <= (obs_r + threshold))
        angle_to_obstacle = atan2(obs_y(i) - y, obs_x(i) - x);
        % Compute the angle difference (normalize to [-pi, pi] range)
        angle_diff=mod(abs(angle_to_obstacle - theta), 2*pi);
        if(abs(angle_diff) <= pi/4)
            obs_flag = 1; % Obstacle detected in front sector
            break;
        else
           obs_flag = 0; 
        end
    end
end
    
if obs_flag && ~obs_flag1
    % Obstacle detected for the first time, trigger recalculation
    recalculate_obs = 1;
else
    % Either no obstacle or already recalculated
    recalculate_obs = 0;
end
x1 = x_d;
y1 = y_d;
theta1 = theta_d;
